simulink library "HybridLibrary"  (R2013a)
settings: Solver=ode45  StartTime=0.0  StopTime=10.0  RelTol=1e-3
values from neighbouring files (symbols this model uses):
  x0 = [10 0 10 0 0]    [mpt3pwacplextst.mat]
undefined symbols (not defined in the file or in its folder): modelReal, TsReal
settings Model: Creator=root  LastModifiedBy=root

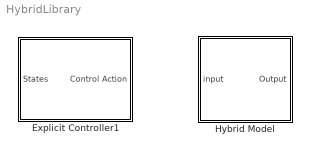
== system HybridLibrary ==
  Explicit Controller1 : Subsystem  mask(MPT Controller){}
      mask help: Evaluates explicit controller for a given state.
      mask Help: Evaluation of an explicit control law is performed by the C-code S-function "mpt_getInput_sfunc", which requires the controller to be exported to C-code using "exportToC".
      mask Display: image(imread('mpt_ctrl.jpg'));
  Hybrid Model : Subsystem

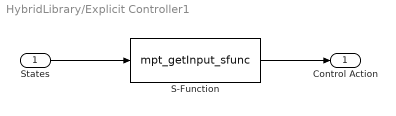
== system HybridLibrary/Explicit Controller1 ==
  States : Inport
  S-Function : S-Function  FunctionName=mpt_getInput_sfunc  EnableBusSupport=off
  Control Action : Outport
  wires:
  States/1 -> S-Function/1
  S-Function/1 -> Control Action/1

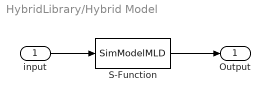
== system HybridLibrary/Hybrid Model ==
  input : Inport
  S-Function : S-Function  FunctionName=SimModelMLD  Parameters=modelReal,x0,TsReal  EnableBusSupport=off
  Output : Outport
  wires:
  input/1 -> S-Function/1
  S-Function/1 -> Output/1
